simulink model "KUKAinv_Dynamics_coupled"  (R2021b)
settings: Solver=ode4  StartTime=0.0  StopTime=0.01  FixedStep=0.01  RelTol=1e-3
InitFcn:
  | % ************** Initiate forces
  | % f0=[0;0;0;0;0;0];
  | % f0=[0;0;0;0;0;0;0];
  | %f_0=[0;0;0];
  | %f_m=[0;1];
  | %f_e=[0;0;0;0;0;0];
  | % ************** Initiate states
  | %q_m=[0;0];
  | %q_dot_m=[0;0];
  | %P=[0;0;0];
  | %V_I0=[0;0;0];
  | % ************** Load main
  | %run(Main.m)
StopFcn:
  | %format long
  | %qddot=out.qddot.data(:,1)
  | %qddot_ref=out.qddot_ref.data(1,:)
values from neighbouring files (symbols this model uses):
  f_0 = [0;0;0;0;0;0]    [Initiate_FQ.m]    (also in Internal_KUKA_Main.m; KUKA_Main.m; Main.m = [0;0;0])
  f_e = [0;0;0;0;0;0]    [Initiate_FQ.m]    (also in Internal_KUKA_Main.m; KUKA_Main.m; Main.m)
  f_m = [0;0.1;0.2;0;0;0.01;0]    [Initiate_FQ.m]    (also in Internal_KUKA_Main.m = [0;0;0;0;0;0;0]; KUKA_Main.m = [0;0;0;0;0;0;0]; Main.m = [0;0])
  I0 = eye(3)*416.667    [Main.m]
  iota0 = eye(6,6)    [Internal_KUKA_Main.m]    (also in KUKA_Main.m; Main.m = [1 0 0; 0 1 0;zeros(3,3);0 0 1])
  m0 = robot.Bodies{1,n+1}.Mass    [Internal_KUKA_Main.m]    (also in KUKA_Main.m; Main.m = 100)
  mm = zeros(1,n)    [Internal_KUKA_Main.m]    (also in KUKA_Main.m; Main.m = [2 2])
  P0 = M0*V_I0+M0\M0m*q_dot_m    [Initiate_FQ.m]    (also in Internal_KUKA_Main.m; KUKA_Main.m)
  q_dot_m = [0;0;0;0;0;0;0]    [Initiate_FQ.m]    (also in Internal_KUKA_Main.m = [qdot1;qdot2;qdot3;qdot4;qdot5;qdot6;qdot7]; KUKA_Main.m = [qdot1;qdot2;qdot3;qdot4;qdot5;qdot6;qdot7]; Main.m = [0;0]; sendJointTorques.m = fread(t, 7, 'double'))
  q_m = [0.2;1.5;0.3;1.8;0.5;0.3;0.6]    [Initiate_FQ.m]    (also in Internal_KUKA_Main.m = [q_m1;q_m2;q_m3;q_m4;q_m5;q_m6;q_m7]; KUKA_Main.m = [q_m1;q_m2;q_m3;q_m4;q_m5;q_m6;q_m7]; Main.m = [0;0]; sendJointTorques.m = fread(t, 7, 'double'))
  sc_size = 0    [Internal_KUKA_Main.m]    (also in KUKA_Main.m = 1)
  V_I0 = [0;0;0;0;0;0]    [Initiate_FQ.m]    (also in Internal_KUKA_Main.m; KUKA_Main.m; Main.m = [0;0;0])
  X = [0 -x(3) x(2) ; x(3) 0 -x(1) ; -x(2) x(1) 0 ]    [skewsym.m]
  Xi_m = Xi_m(1:robot.n*6,1:robot.n)    [Internal_KUKA_Main.m]    (also in KUKA_Main.m)
  Xi_m_matrix = zeros(6*n,n)    [Internal_KUKA_Main.m]    (also in KUKA_Main.m; Main.m)
undefined symbols (not defined in the file or in its folder): g_cm, g_cm0, Im, m0_frak, m_diag, Y, Z
libraries: sm_lib x47, nesl_utility x41, robotcorelib x1
(part 1 of 2)
settings Model: Creator=Bmmog  LastModifiedBy=Bmmog
settings SimscapeCC: SimscapeLogType=all  SimscapeLogSimulationStatistics=on

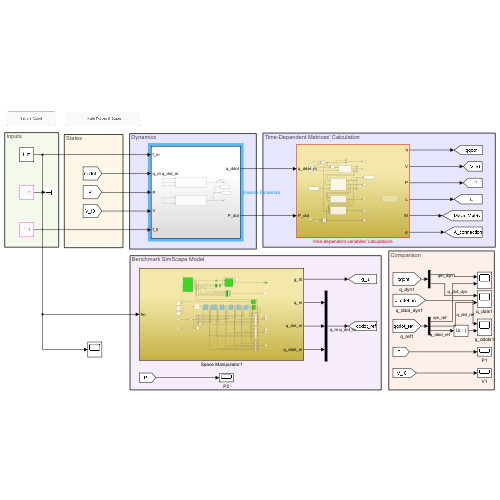
[thumbnail: Simulink's stored preview of the top-level diagram]
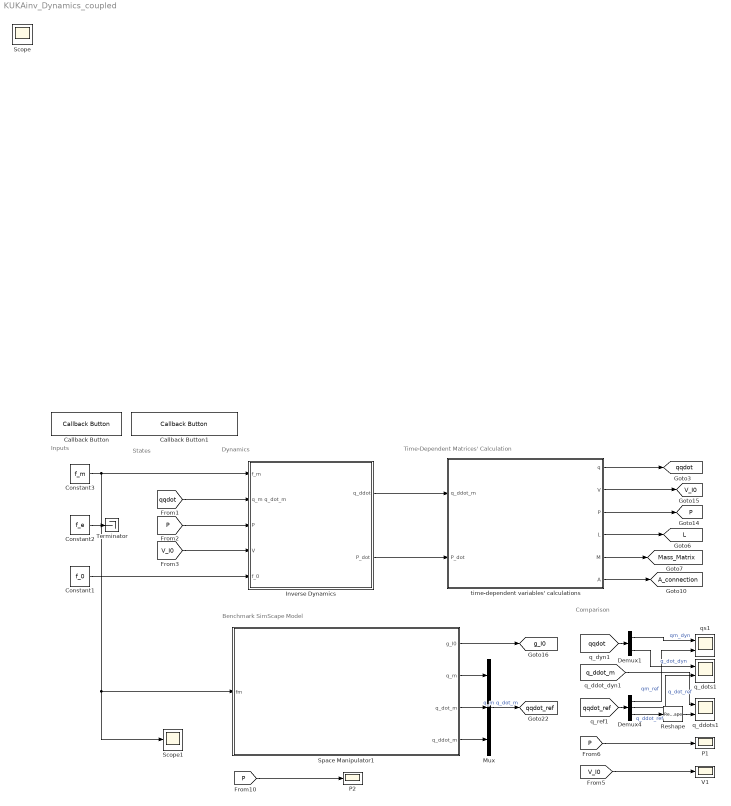
== system KUKAinv_Dynamics_coupled ==
  note: Dynamics
  note: Time-Dependent Matrices' Calculation
  note: States
  note: Comparison
  note: Inputs
  note: Benchmark SimScape Model
  Callback Button : CallbackButton  ButtonText=Initiate Robot
      settings: ClickFcn=Initiate_KUKA_inv
  Callback Button1 : CallbackButton  ButtonText=Initiate Forces & States
      settings: ClickFcn=Initiate_FQ
  Constant1 : Constant  Value=f_0  VectorParams1D=off
  Constant2 : Constant  Value=f_e  VectorParams1D=off
  Constant3 : Constant  Value=f_m  VectorParams1D=off
  Demux1 : Demux  Outputs=2
  Demux4 : Demux  Outputs=[7 7 7]
  Inverse Dynamics : Subsystem
  Mux : Mux  Inputs=3
  P1 : Scope
  P2 : Scope
  Reshape : Reshape
  Scope1 : Scope
  Space Manipulator1 : Subsystem
  Terminator : Terminator
  V1 : Scope
  q_ddots1 : Scope  NumInputPorts=2
  q_dots1 : Scope  NumInputPorts=2
  qs1 : Scope  NumInputPorts=2
  time-dependent variables' calculations : Subsystem
  Scope : Scope
  tag scope: A_connection=global, L=global, Mass_Matrix=global, P=global, V_I0=global, g_I0=global, qqdot=global, qqdot_ref=global
  wires:
  Demux4/3 -> Reshape/1  "q_ddot_ref"
  [qqdot] -> Inverse Dynamics/2(q_m q_dot_m)
  [qqdot_ref] -> Demux4/1
  Demux4/1 -> qs1/2  "qm_ref"
  Demux4/2 -> q_dots1/2  "q_dot_ref"
  [qqdot] -> Demux1/1
  Inverse Dynamics/1(q_ddot) -> time-dependent variables' calculations/1(q_ddot_m)
  Demux1/2 -> q_dots1/1  "q_dot_dyn"
  time-dependent variables' calculations/4(L) -> [L]
  time-dependent variables' calculations/5(M) -> [Mass_Matrix]
  time-dependent variables' calculations/1(q) -> [qqdot]
  Demux1/1 -> qs1/1  "qm_dyn"
  time-dependent variables' calculations/6(A) -> [A_connection]
  time-dependent variables' calculations/3(P) -> [P]
  time-dependent variables' calculations/2(V) -> [V_I0]
  Inverse Dynamics/2(P_dot) -> time-dependent variables' calculations/2(P_dot)
  [P] -> Inverse Dynamics/3(P)
  [V_I0] -> Inverse Dynamics/4(V)
  Constant1/1 -> Inverse Dynamics/5(f_0)
  [P] -> P1/1
  [V_I0] -> V1/1
  Space Manipulator1/3(q_dot_m) -> Mux/2
  Space Manipulator1/1(g_I0) -> [g_I0]
  Mux/1 -> [qqdot_ref]  "q_m q_dot_m"
  [P] -> P2/1
  Space Manipulator1/2(q_m) -> Mux/1
  Space Manipulator1/4(q_ddot_m) -> Mux/3
  Constant2/1 -> Terminator/1
  Constant3/1 -> Space Manipulator1/1(fm), Scope1/1, Inverse Dynamics/1(f_m)
  [q_ddot_m] -> q_ddots1/1
  Reshape/1 -> q_ddots1/2

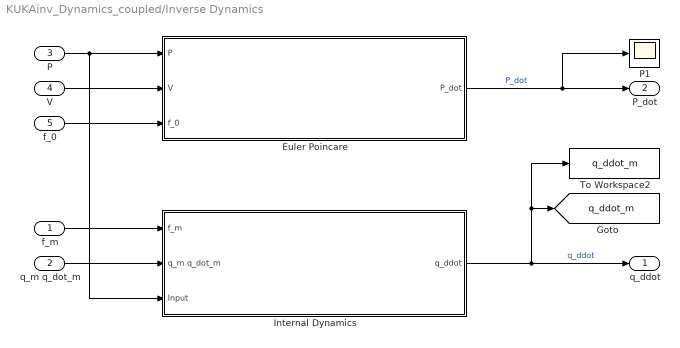
== system KUKAinv_Dynamics_coupled/Inverse Dynamics ==
  f_m : Inport
  q_m q_dot_m : Inport  Port=2
  P : Inport  Port=3
  V : Inport  Port=4
  f_0 : Inport  Port=5
  Euler Poincare : Subsystem
  Internal Dynamics : Subsystem
  P1 : Scope
  To Workspace2 : ToWorkspace  VariableName=q_ddot_m  SaveFormat=Timeseries  SampleTime=-1
  q_ddot : Outport
  P_dot : Outport  Port=2
  tag scope: q_ddot_m=global
  wires:
  f_m/1 -> Internal Dynamics/1(f_m)
  Internal Dynamics/1(q_ddot) -> To Workspace2/1, [q_ddot_m], q_ddot/1  "q_ddot"
  q_m q_dot_m/1 -> Internal Dynamics/2(q_m q_dot_m)
  Euler Poincare/1(P_dot) -> P1/1, P_dot/1  "P_dot"
  V/1 -> Euler Poincare/2(V)
  f_0/1 -> Euler Poincare/3(f_0)
  P/1 -> Internal Dynamics/3(Input), Euler Poincare/1(P)

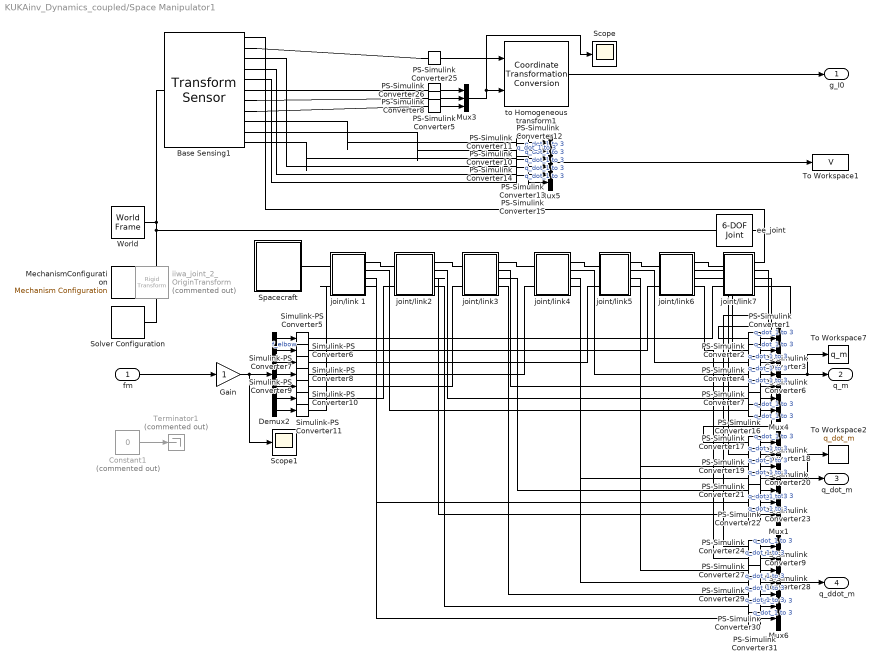
== system KUKAinv_Dynamics_coupled/Space Manipulator1 ==
  fm : Inport
  Base Sensing1 : sm_lib/Frames and Transforms/Transform Sensor  MeasurementFrame=Base  SenseAngle=off  SenseAxis=off  SenseAngle1=off  SenseAngle2=off  SenseAngle3=off  SenseQ=off  SenseR=on  SenseOmegaX=on  SenseOmegaY=on  SenseOmegaZ=on  SenseOmega1=off  SenseOmega2=off  SenseOmega3=off  SenseQDot=off  SenseRDot=off  SenseAlphaX=off  SenseAlphaY=off  SenseAlphaZ=off  SenseAlpha1=off  SenseAlpha2=off  SenseAlpha3=off  SenseQDDot=off  SenseRDDot=off  SenseX=on  SenseY=on  SenseZ=on  SenseRad=off  SenseAzim=off  SenseDist=off  SenseInc=off  SenseXDot=on  SenseYDot=on  SenseZDot=on  SenseRadDot=off  SenseAzimDot=off  SenseDistDot=off  SenseIncDot=off  SenseXDDot=off  SenseYDDot=off  SenseZDDot=off  SenseRadDDot=off  SenseAzimDDot=off  SenseDistDDot=off  SenseIncDDot=off
  Constant1 : Constant  Commented=on  Value=0
  Demux2 : Demux  Outputs=7
  Gain : Gain
  MechanismConfiguration : sm_lib/Utilities/Mechanism Configuration  UniformGravity=None  GravityVector=[0 0 0]  GravityUnits=m/s^2  LinearizationDelta=0.001  JointModeTransitionNonlinearIterations=2
  Mux1 : Mux  Inputs=7
  Mux3 : Mux  Inputs=3
  Mux4 : Mux  Inputs=7
  Mux5 : Mux  Inputs=6
  Mux6 : Mux  Inputs=7
  PS-Simulink Converter{1..31} (31 alike) : nesl_utility/PS-Simulink Converter  PhysicalDomain=network_engine_domain  SubClassName=ps_output  LeftPortType=input  RightPortType=output  PseudoPeriodic=off  Frequencies=[]  Unit=inherit  AffineConversion=off
      settings: SourceProductBaseCode=PW,SS
  Scope : Scope
  Scope1 : Scope
  Simulink-PS Converter{5..11} (7 alike) : nesl_utility/Simulink-PS Converter  PhysicalDomain=network_engine_domain  SubClassName=ps_input  LeftPortType=input  RightPortType=output  PseudoPeriodic=off  Frequencies=[]  NoiseDistribution=none  NoiseParameters=[]  Unit=1  AffineConversion=off  FilteringAndDerivatives=provide  SimscapeFilterOrder=1  InputFilterTimeConstant=0.001  UdotUserProvided=0
      settings: SourceProductBaseCode=PW,SS
  Solver Configuration : nesl_utility/Solver Configuration  PhysicalDomain=network_engine_domain  SubClassName=solver  LeftPortType=input  RightPortType=generic  Tones=[]  Harmonics=[]  SimulateNoise=off  Profile=off  UseLocalSampling=off  EnableSwitchedLinearOptims=on  FrequencyDomain=off  UseCCode=off  RelTol=0.001  AbsTol=0.001  MinStep=1e-09  ToWorkspace=off  RevertToSquareIcSolve=off  NumHomotopyIterations=100  PhasorMode=off  PhasorModeNumHarmonics=1  DoDC=off  ResidualTolerance=1e-09  UseLocalSolver=on  LocalSolverChoice=NE_BACKWARD_EULER_ADVANCER  LocalSolverSampleTime=0.001  DoFixedCost=on  MaxNonlinIter=3  MaxModeIter=2  ComputeImpulses=off  ImpulseIterations=2  LinearAlgebra=auto  EquationFormulation=NE_TIME_EF  DelaysMemoryBudget=1024  AutomaticFiltering=on  FilteringTimeConstant=0.001  PartitionStorageMethod=AS_NEEDED  PartitionMemoryBudget=1024  PartitionMethod=ROBUST
      settings: SourceProductBaseCode=PW,SS
  Spacecraft : Subsystem
  Terminator1 : Terminator  Commented=on
  To Workspace1 : ToWorkspace  VariableName=V  SaveFormat=Timeseries  SampleTime=-1
  To Workspace2 : ToWorkspace  VariableName=q_dot_m  SampleTime=-1
  To Workspace7 : ToWorkspace  VariableName=q_m  SampleTime=-1
  World : sm_lib/Frames and Transforms/World Frame
  ee_joint : sm_lib/Joints/6-DOF Joint  JointMode=Normal  SenseConstraintForce=off  SenseConstraintForceX=off  SenseConstraintForceY=off  SenseConstraintForceZ=off  SenseConstraintTorque=off  SenseConstraintTorqueX=off  SenseConstraintTorqueY=off  SenseConstraintTorqueZ=off  SenseTotalForce=off  SenseTotalForceX=off  SenseTotalForceY=off  SenseTotalForceZ=off  SenseTotalTorque=off  SenseTotalTorqueX=off  SenseTotalTorqueY=off  SenseTotalTorqueZ=off  CompositeWrenchDir=FollowerOnBase  CompositeWrenchFrame=BaseFrame  PxEquilibriumPosition=0  PxEquilibriumPositionUnits=m  PxSpringStiffness=0  PxSpringStiffnessUnits=N/m  PxDampingCoefficient=0  PxDampingCoefficientUnits=N/(m/s)  PxTorqueActuationMode=NoTorque  PxMotionActuationMode=ComputedMotion  PxSensePosition=off  PxSenseVelocity=off  PxSenseAcceleration=off  PxSenseTorqueForce=off  PxSenseLowerLimitTorqueForce=off  PxSenseUpperLimitTorqueForce=off  PxLowerLimitSpecify=off  PxLowerLimitBound=-1  PxLowerLimitBoundUnits=m  PxLowerLimitStiffness=1e6  PxLowerLimitStiffnessUnits=N/m  PxLowerLimitDamping=1e3  PxLowerLimitDampingUnits=N/(m/s)  PxLowerLimitTransitionRegionWidth=1e-4  PxLowerLimitTransitionRegionWidthUnits=m  PxUpperLimitSpecify=off  PxUpperLimitBound=1  PxUpperLimitBoundUnits=m  PxUpperLimitStiffness=1e6  PxUpperLimitStiffnessUnits=N/m  PxUpperLimitDamping=1e3  PxUpperLimitDampingUnits=N/(m/s)  PxUpperLimitTransitionRegionWidth=1e-4  PxUpperLimitTransitionRegionWidthUnits=m  PxPositionTargetSpecify=off  PxPositionTargetPriority=High  PxPositionTargetValue=0  PxPositionTargetValueUnits=m  PxVelocityTargetSpecify=on  PxVelocityTargetPriority=High  PxVelocityTargetValue=V_I0(1)  PxVelocityTargetValueUnits=m/s  PyEquilibriumPosition=0  PyEquilibriumPositionUnits=m  PySpringStiffness=0  PySpringStiffnessUnits=N/m  PyDampingCoefficient=0  PyDampingCoefficientUnits=N/(m/s)  PyTorqueActuationMode=NoTorque  PyMotionActuationMode=ComputedMotion  PySensePosition=off  PySenseVelocity=off  PySenseAcceleration=off  PySenseTorqueForce=off  PySenseLowerLimitTorqueForce=off  PySenseUpperLimitTorqueForce=off  PyLowerLimitSpecify=off  PyLowerLimitBound=-1  PyLowerLimitBoundUnits=m  PyLowerLimitStiffness=1e6  PyLowerLimitStiffnessUnits=N/m  PyLowerLimitDamping=1e3  PyLowerLimitDampingUnits=N/(m/s)  PyLowerLimitTransitionRegionWidth=1e-4  PyLowerLimitTransitionRegionWidthUnits=m  PyUpperLimitSpecify=off  PyUpperLimitBound=1  PyUpperLimitBoundUnits=m  PyUpperLimitStiffness=1e6  PyUpperLimitStiffnessUnits=N/m  PyUpperLimitDamping=1e3  PyUpperLimitDampingUnits=N/(m/s)  PyUpperLimitTransitionRegionWidth=1e-4  PyUpperLimitTransitionRegionWidthUnits=m  PyPositionTargetSpecify=off  PyPositionTargetPriority=High  PyPositionTargetValue=0  PyPositionTargetValueUnits=m  PyVelocityTargetSpecify=on  PyVelocityTargetPriority=High  PyVelocityTargetValue=V_I0(2)  PyVelocityTargetValueUnits=m/s  PzEquilibriumPosition=0  PzEquilibriumPositionUnits=m  PzSpringStiffness=0  PzSpringStiffnessUnits=N/m  PzDampingCoefficient=0  PzDampingCoefficientUnits=N/(m/s)  PzTorqueActuationMode=NoTorque  PzMotionActuationMode=ComputedMotion  PzSensePosition=off  PzSenseVelocity=off  PzSenseAcceleration=off  PzSenseTorqueForce=off  PzSenseLowerLimitTorqueForce=off  PzSenseUpperLimitTorqueForce=off  PzLowerLimitSpecify=off  PzLowerLimitBound=-1  PzLowerLimitBoundUnits=m  PzLowerLimitStiffness=1e6  PzLowerLimitStiffnessUnits=N/m  PzLowerLimitDamping=1e3  PzLowerLimitDampingUnits=N/(m/s)  PzLowerLimitTransitionRegionWidth=1e-4  PzLowerLimitTransitionRegionWidthUnits=m  PzUpperLimitSpecify=off  PzUpperLimitBound=1  PzUpperLimitBoundUnits=m  PzUpperLimitStiffness=1e6  PzUpperLimitStiffnessUnits=N/m  PzUpperLimitDamping=1e3  PzUpperLimitDampingUnits=N/(m/s)  PzUpperLimitTransitionRegionWidth=1e-4  PzUpperLimitTransitionRegionWidthUnits=m  PzPositionTargetSpecify=off  PzPositionTargetPriority=High  PzPositionTargetValue=0  PzPositionTargetValueUnits=m  PzVelocityTargetSpecify=on  PzVelocityTargetPriority=High  PzVelocityTargetValue=V_I0(3)  PzVelocityTargetValueUnits=m/s  SphDefPosRotationMethod=None  SphDefPosRotationAngleUnits=deg  SphDefPosRotationStandardAxis=+Z  SphDefPosRotationAngle=0.0  SphDefPosRotationArbitraryAxis=[0 0 1]  SphDefPosFollAlignAxisA=+X  SphDefPosBaseAlignAxisA=+Y  SphDefPosFollAlignAxisB=+Y  SphDefPosBaseAlignAxisB=+Z  SphDefPosRotationSequenceAxes=FollowerAxes  SphDefPosRotationSequence=XYX  SphDefPosRotationSequenceAngles=[0 0 0]  SphDefPosRotationSequenceAnglesUnits=deg  SphDefPosRotationMatrix=[1 0 0; 0 1 0; 0 0 1]  SphEqPosRotationMethod=None  SphEqPosRotationAngleUnits=deg  SphEqPosRotationStandardAxis=+Z  SphEqPosRotationAngle=0.0  SphEqPosRotationArbitraryAxis=[0 0 1]  SphEqPosFollAlignAxisA=+X  SphEqPosBaseAlignAxisA=+Y  SphEqPosFollAlignAxisB=+Y  SphEqPosBaseAlignAxisB=+Z  SphEqPosRotationSequenceAxes=FollowerAxes  SphEqPosRotationSequence=XYX  SphEqPosRotationSequenceAngles=[0 0 0]  SphEqPosRotationSequenceAnglesUnits=deg  SphEqPosRotationMatrix=[1 0 0; 0 1 0; 0 0 1]  SphSpringStiffness=0  SphSpringStiffnessUnits=N*m/deg  SphDampingCoefficient=0  SphDampingCoefficientUnits=N*m/(deg/s)  SphActuateTorqueX=off  SphActuateTorqueY=off  SphActuateTorqueZ=off  SphActuateTorque=off  SphTorqueActuationMode=NoTorque  SphMotionActuationMode=ComputedMotion  SphActuationFrame=BaseFrame  SphSensePosition=off  SphSenseVelocityX=off  SphSenseVelocityY=off  SphSenseVelocityZ=off  SphSenseVelocity=off  SphSenseAccelerationX=off  SphSenseAccelerationY=off  SphSenseAccelerationZ=off  SphSenseAcceleration=off  SphSenseTorqueX=off  SphSenseTorqueY=off  SphSenseTorqueZ=off  SphSenseTorqueForce=off  SphSenseLowerLimitTorqueMag=off  SphSenseUpperLimitTorqueMag=off  SphSensingFrame=BaseFrame  SphLowerLimitSpecify=off  SphLowerLimitBound=15  SphLowerLimitBoundUnits=deg  SphLowerLimitStiffness=1e4  SphLowerLimitStiffnessUnits=N*m/deg  SphLowerLimitDamping=10  SphLowerLimitDampingUnits=N*m/(deg/s)  SphLowerLimitTransitionRegionWidth=0.1  SphLowerLimitTransitionRegionWidthUnits=deg  SphUpperLimitSpecify=off  SphUpperLimitBound=45  SphUpperLimitBoundUnits=deg  SphUpperLimitStiffness=1e4  SphUpperLimitStiffnessUnits=N*m/deg  SphUpperLimitDamping=10  SphUpperLimitDampingUnits=N*m/(deg/s)  SphUpperLimitTransitionRegionWidth=0.1  SphUpperLimitTransitionRegionWidthUnits=deg  SphPositionTargetRotationMethod=RotationSequence  SphPositionTargetRotationAngleUnits=deg  SphPositionTargetRotationStandardAxis=+Z  SphPositionTargetRotationAngle=0.0  SphPositionTargetRotationArbitraryAxis=[0 0 1]  SphPositionTargetFollAlignAxisA=+X  SphPositionTargetBaseAlignAxisA=+Y  SphPositionTargetFollAlignAxisB=+Y  SphPositionTargetBaseAlignAxisB=+Z  SphPositionTargetRotationSequenceAxes=FollowerAxes  SphPositionTargetRotationSequence=ZYX  SphPositionTargetRotationSequenceAngles=[0 0 0]  SphPositionTargetRotationSequenceAnglesUnits=deg  SphPositionTargetRotationMatrix=[1 0 0; 0 1 0; 0 0 1]  SphPositionTargetSpecify=off  SphPositionTargetPriority=High  SphVelocityTargetValue=[V_I0(4) V_I0(5) V_I0(6)]  SphVelocityTargetValueUnits=rad/s  SphVelocityTargetSpecify=on  SphVelocityTargetPriority=High  SphVelocityTargetInFollowerFrame=on
  iiwa_joint_2_OriginTransform : sm_lib/Frames and Transforms/Rigid Transform  Commented=on  TranslationMethod=Cartesian  TranslationStandardOffset=0  TranslationLengthUnit=m  TranslationStandardAxis=+Z  TranslationCartesianOffset=g_cm(1:3,4,7)'  TranslationROffset=0  TranslationROffsetUnits=m  TranslationZOffset=0  TranslationZOffsetUnits=m  TranslationThetaOffset=0  TranslationThetaOffsetUnits=deg  RotationMethod=RotationMatrix  RotationAngleUnits=deg  RotationStandardAxis=+Z  RotationAngle=0.0  RotationArbitraryAxis=[0 0 1]  FollAlignAxisA=+X  BaseAlignAxisA=+Y  FollAlignAxisB=+Y  BaseAlignAxisB=+Z  RotationSequenceAxes=BaseAxes  RotationSequence=XYZ  RotationSequenceAngles=[1.57079632679, 0, 3.14159265359]  RotationSequenceAnglesUnits=rad  RotationMatrix=g_cm(1:3,1:3,7)
  join/link 1 : Subsystem
  joint/link2 : Subsystem
  joint/link3 : Subsystem
  joint/link4 : Subsystem
  joint/link5 : Subsystem
  joint/link6 : Subsystem
  joint/link7 : Subsystem
  to Homogeneous transform1 : robotcorelib/Coordinate Transformation Conversion  InputRepresentation=Rotation Matrix  InputEulerSequence=ZYX  ShowTrVecInputPort=on  OutputRepresentation=Homogeneous Transformation  OutputEulerSequence=ZYX  ShowTrVecOutputPort=on  SimulateUsing=Interpreted execution
      settings: SourceProductBaseCode=NV,RO,RR,UV
  g_I0 : Outport
  q_m : Outport  Port=2
  q_dot_m : Outport  Port=3
  q_ddot_m : Outport  Port=4
  wires:
  Demux2/1 -> Simulink-PS Converter5/1
  Demux2/3 -> Simulink-PS Converter7/1
  PS-Simulink Converter15/1 -> Mux5/6  "q_dot_1 to 3"
  PS-Simulink Converter10/1 -> Mux5/3  "q_dot_1 to 3"
  fm/1 -> Gain/1
  PS-Simulink Converter25/1 -> to Homogeneous transform1/1
  Gain/1 -> Scope1/1, Demux2/1
  Mux5/1 -> To Workspace1/1
  PS-Simulink Converter8/1 -> Mux3/3
  Mux3/1 -> Scope/1, to Homogeneous transform1/2
  PS-Simulink Converter12/1 -> Mux5/2  "q_dot_1 to 3"
  to Homogeneous transform1/1 -> g_I0/1
  PS-Simulink Converter13/1 -> Mux5/4  "q_dot_1 to 3"
  PS-Simulink Converter26/1 -> Mux3/1
  Demux2/7 -> Simulink-PS Converter11/1
  PS-Simulink Converter14/1 -> Mux5/5  "q_dot_1 to 3"
  Demux2/4 -> Simulink-PS Converter8/1
  PS-Simulink Converter11/1 -> Mux5/1  "q_dot_1 to 3"
  PS-Simulink Converter5/1 -> Mux3/2
  Demux2/6 -> Simulink-PS Converter10/1
  Constant1/1 -> Terminator1/1
  Demux2/2 -> Simulink-PS Converter6/1  "f_elbow"
  Demux2/5 -> Simulink-PS Converter9/1
  PS-Simulink Converter27/1 -> Mux6/3  "q_dot_1 to 3"
  PS-Simulink Converter1/1 -> Mux4/1  "q_dot_1 to 3"
  PS-Simulink Converter6/1 -> Mux4/5  "q_dot_1 to 3"
  PS-Simulink Converter30/1 -> Mux6/6  "q_dot_1 to 3"
  PS-Simulink Converter3/1 -> Mux4/3  "q_dot_1 to 3"
  PS-Simulink Converter18/1 -> Mux1/2  "q_dot_1 to 3"
  PS-Simulink Converter31/1 -> Mux6/7  "q_dot_1 to 3"
  PS-Simulink Converter9/1 -> Mux6/2  "q_dot_1 to 3"
  PS-Simulink Converter7/1 -> Mux4/6  "q_dot_1 to 3"
  PS-Simulink Converter2/1 -> Mux4/2  "q_dot_1 to 3"
  PS-Simulink Converter4/1 -> Mux4/4  "q_dot_1 to 3"
  PS-Simulink Converter21/1 -> Mux1/5  "q_dot_1 to 3"
  PS-Simulink Converter23/1 -> Mux1/7  "q_dot_1 to 3"
  PS-Simulink Converter16/1 -> Mux4/7  "q_dot_1 to 3"
  PS-Simulink Converter28/1 -> Mux6/4  "q_dot_1 to 3"
  Mux4/1 -> q_m/1, To Workspace7/1
  Mux1/1 -> q_dot_m/1, To Workspace2/1
  PS-Simulink Converter24/1 -> Mux6/1  "q_dot_1 to 3"
  Mux6/1 -> q_ddot_m/1
  PS-Simulink Converter20/1 -> Mux1/4  "q_dot_1 to 3"
  PS-Simulink Converter29/1 -> Mux6/5  "q_dot_1 to 3"
  PS-Simulink Converter22/1 -> Mux1/6  "q_dot_1 to 3"
  PS-Simulink Converter17/1 -> Mux1/1  "q_dot_1 to 3"
  PS-Simulink Converter19/1 -> Mux1/3  "q_dot_1 to 3"
  connections:
  ee_joint/LConn1 -- MechanismConfiguration/RConn1 -- Solver Configuration/RConn1 -- World/RConn1 -- Base Sensing1/LConn1
  ee_joint/RConn1 -- Base Sensing1/RConn1 -- joint/link7/RConn1
  joint/link4/LConn1 -- joint/link3/RConn1
  Base Sensing1/RConn10 -- PS-Simulink Converter12/LConn1
  Simulink-PS Converter9/RConn1 -- joint/link3/LConn2
  Simulink-PS Converter8/RConn1 -- joint/link4/LConn2
  Base Sensing1/RConn2 -- PS-Simulink Converter25/LConn1
  joint/link5/LConn1 -- joint/link4/RConn1
  Base Sensing1/RConn5 -- PS-Simulink Converter15/LConn1
  Base Sensing1/RConn7 -- PS-Simulink Converter5/LConn1
  joint/link6/LConn1 -- joint/link5/RConn1
  Base Sensing1/RConn11 -- PS-Simulink Converter10/LConn1
  Base Sensing1/RConn3 -- PS-Simulink Converter13/LConn1
  Simulink-PS Converter5/RConn1 -- joint/link7/LConn2
  Base Sensing1/RConn4 -- PS-Simulink Converter14/LConn1
  Base Sensing1/RConn9 -- PS-Simulink Converter11/LConn1
  Base Sensing1/RConn8 -- PS-Simulink Converter8/LConn1
  Base Sensing1/RConn6 -- PS-Simulink Converter26/LConn1
  Simulink-PS Converter7/RConn1 -- joint/link5/LConn2
  joint/link6/RConn3 -- PS-Simulink Converter18/LConn1
  joint/link6/RConn4 -- PS-Simulink Converter9/LConn1
  joint/link5/RConn2 -- PS-Simulink Converter3/LConn1
  joint/link5/RConn3 -- PS-Simulink Converter19/LConn1
  joint/link5/RConn4 -- PS-Simulink Converter27/LConn1
  joint/link4/RConn2 -- PS-Simulink Converter4/LConn1
  joint/link4/RConn3 -- PS-Simulink Converter20/LConn1
  joint/link4/RConn4 -- PS-Simulink Converter28/LConn1
  joint/link3/RConn2 -- PS-Simulink Converter6/LConn1
  joint/link3/RConn3 -- PS-Simulink Converter21/LConn1
  joint/link3/RConn4 -- PS-Simulink Converter29/LConn1
  joint/link6/RConn1 -- joint/link7/LConn1
  joint/link6/RConn2 -- PS-Simulink Converter2/LConn1
  joint/link6/LConn2 -- Simulink-PS Converter6/RConn1
  joint/link7/RConn2 -- PS-Simulink Converter1/LConn1
  joint/link7/RConn3 -- PS-Simulink Converter17/LConn1
  joint/link7/RConn4 -- PS-Simulink Converter24/LConn1
  join/link 1/LConn2 -- Simulink-PS Converter11/RConn1
  join/link 1/LConn1 -- Spacecraft/RConn1
  join/link 1/RConn1 -- joint/link2/LConn1
  Simulink-PS Converter10/RConn1 -- joint/link2/LConn2
  joint/link3/LConn1 -- joint/link2/RConn1
  join/link 1/RConn2 -- PS-Simulink Converter16/LConn1
  joint/link2/RConn3 -- PS-Simulink Converter23/LConn1
  PS-Simulink Converter7/LConn1 -- joint/link2/RConn2
  join/link 1/RConn3 -- PS-Simulink Converter22/LConn1
  joint/link2/RConn4 -- PS-Simulink Converter30/LConn1
  join/link 1/RConn4 -- PS-Simulink Converter31/LConn1

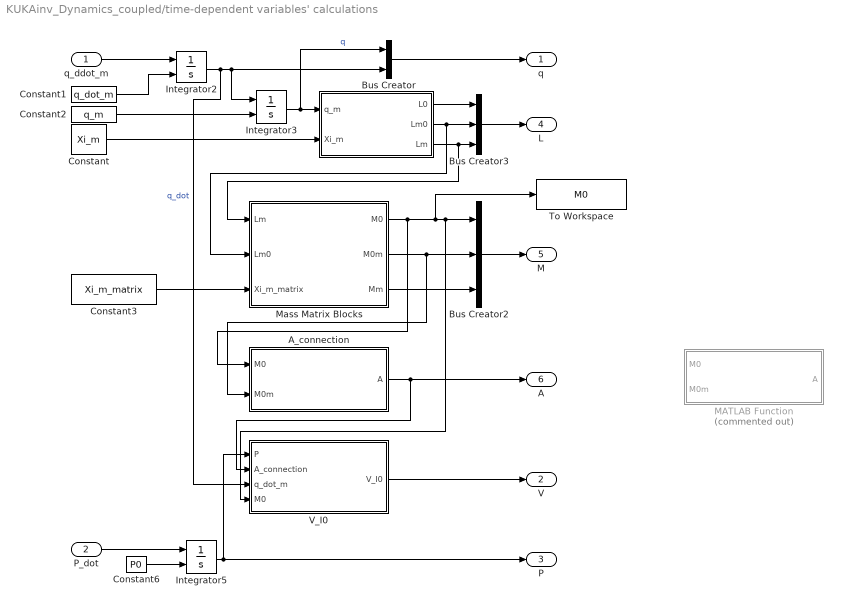
== system KUKAinv_Dynamics_coupled/time-dependent variables' calculations ==
  q_ddot_m : Inport
  P_dot : Inport  Port=2
  " " : MATLAB Function  TreatAsAtomicUnit=on
  A_connection : Subsystem
  Bus Creator : BusCreator  Inputs=2
  Bus Creator2 : BusCreator  Inputs=3
  Bus Creator3 : BusCreator  Inputs=3
  Constant : Constant  Value=Xi_m
  Constant1 : Constant  Value=q_dot_m  VectorParams1D=off
  Constant2 : Constant  Value=q_m  VectorParams1D=off
  Constant3 : Constant  Value=Xi_m_matrix
  Constant6 : Constant  Value=P0  VectorParams1D=off
  Integrator2 : Integrator  InitialConditionSource=external  InitialCondition=q_dot_m
  Integrator3 : Integrator  InitialConditionSource=external
  Integrator5 : Integrator  InitialConditionSource=external  ContinuousStateAttributes='momentum'
  MATLAB Function : MATLAB Function  Commented=on  TreatAsAtomicUnit=on
  Mass Matrix Blocks : Subsystem
  To Workspace : ToWorkspace  VariableName=M0  SaveFormat=Timeseries  SampleTime=-1
  V_I0 : MATLAB Function  TreatAsAtomicUnit=on
  q : Outport
  V : Outport  Port=2
  P : Outport  Port=3
  L : Outport  Port=4
  M : Outport  Port=5
  A : Outport  Port=6
  wires:
  q_ddot_m/1 -> Integrator2/1
  " "/3(Lm) -> Bus Creator3/3, Mass Matrix Blocks/1(Lm)
  Constant3/1 -> Mass Matrix Blocks/3(Xi_m_matrix)
  Constant/1 -> " "/2(Xi_m)
  Constant1/1 -> Integrator2/2
  Constant2/1 -> Integrator3/2
  Bus Creator/1 -> q/1
  Integrator3/1 -> Bus Creator/1, " "/1(q_m)  "q"
  Integrator2/1 -> V_I0/3(q_dot_m), Bus Creator/2, Integrator3/1  "q_dot"
  V_I0/1(V_I0) -> V/1
  Integrator5/1 -> V_I0/1(P), P/1
  P_dot/1 -> Integrator5/1
  Constant6/1 -> Integrator5/2
  Mass Matrix Blocks/3(Mm) -> Bus Creator2/3
  " "/2(Lm0) -> Mass Matrix Blocks/2(Lm0), Bus Creator3/2
  " "/1(L0) -> Bus Creator3/1
  Bus Creator3/1 -> L/1
  Bus Creator2/1 -> M/1
  Mass Matrix Blocks/1(M0) -> A_connection/1(M0), To Workspace/1, V_I0/4(M0), Bus Creator2/1
  Mass Matrix Blocks/2(M0m) -> A_connection/2(M0m), Bus Creator2/2
  A_connection/1(A) -> V_I0/2(A_connection), A/1

== system KUKAinv_Dynamics_coupled/Inverse Dynamics/Euler Poincare ==
  P : Inport
  V : Inport  Port=2
  f_0 : Inport  Port=3
  Add : Sum
  Constant1 : Constant  Commented=on  Value=eye(6,6)
  MATLAB Function : MATLAB Function  Commented=on  TreatAsAtomicUnit=on
  Matrix Multiply : Product  Multiplication=Matrix(*)
  adj_low_tilde : MATLAB Function  TreatAsAtomicUnit=on
  P_dot : Outport
  wires:
  P/1 -> adj_low_tilde/1(P)
  V/1 -> Matrix Multiply/2
  Matrix Multiply/1 -> Add/1
  f_0/1 -> Add/2
  Add/1 -> P_dot/1
  adj_low_tilde/1(adj_low_tilde) -> Matrix Multiply/1

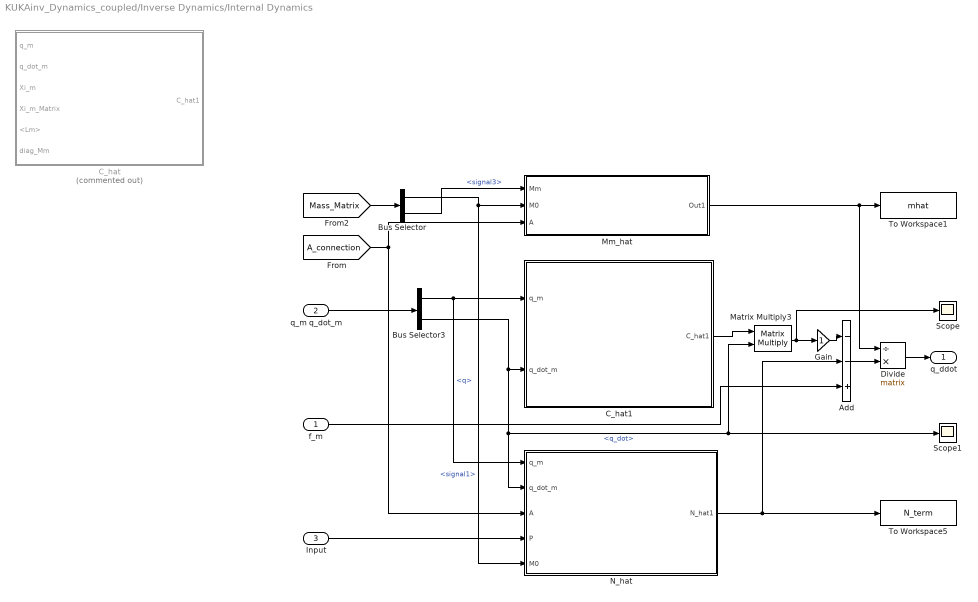
== system KUKAinv_Dynamics_coupled/Inverse Dynamics/Internal Dynamics ==
  f_m : Inport
  q_m q_dot_m : Inport  Port=2
  Input : Inport  Port=3
  Add : Sum  Inputs=--+
  Bus Selector : BusSelector  OutputSignals=signal1,signal3
  Bus Selector3 : BusSelector  OutputSignals=q,q_dot
  C_hat : Subsystem  Commented=on
  C_hat1 : Subsystem
  Divide : Product  Inputs=/*  Multiplication=Matrix(*)
  Gain : Gain
  Matrix Multiply3 : Product  Multiplication=Matrix(*)
  Mm_hat : Subsystem
  N_hat : Subsystem
  Scope : Scope
  Scope1 : Scope
  To Workspace1 : ToWorkspace  VariableName=mhat  SaveFormat=Timeseries  SampleTime=-1
  To Workspace5 : ToWorkspace  VariableName=N_term  SaveFormat=Timeseries  SampleTime=-1
  q_ddot : Outport
  wires:
  f_m/1 -> Add/3
  C_hat1/1(C_hat1) -> Matrix Multiply3/1
  Matrix Multiply3/1 -> Scope/1, Gain/1
  Bus Selector3/2 -> N_hat/2(q_dot_m), Scope1/1, Matrix Multiply3/2, C_hat1/2(q_dot_m)  "<q_dot>"
  q_m q_dot_m/1 -> Bus Selector3/1
  Divide/1 -> q_ddot/1
  Bus Selector3/1 -> N_hat/1(q_m), C_hat1/1(q_m)  "<q>"
  Add/1 -> Divide/2
  [Mass_Matrix] -> Bus Selector/1
  Gain/1 -> Add/1
  Bus Selector/1 -> N_hat/5(M0), Mm_hat/2(M0)  "<signal1>"
  [A_connection] -> Mm_hat/3(A), N_hat/3(A)
  Input/1 -> N_hat/4(P)
  N_hat/1(N_hat1) -> To Workspace5/1, Add/2
  Mm_hat/1(Out1) -> Divide/1, To Workspace1/1
  Bus Selector/2 -> Mm_hat/1(Mm)  "<signal3>"

== system KUKAinv_Dynamics_coupled/Space Manipulator1/Spacecraft ==
  Base1 : sm_lib/Body Elements/Brick Solid  GraphicAmbientColor=[0.15 0.15 0.15 1.0]  BasedOnType=Mass  BrickDimensions=[sc_size,sc_size,sc_size]  BrickDimensionUnits=m  CenterOfMass=[0 0 0]  CenterOfMassUnits=m  GraphicDiffuseColor=[0.5 0.5 0.5]  Density=1000  DensityUnits=kg/m^3  DoExposeReferenceFrame=on  GraphicEmissiveColor=[0.0 0.0 0.0 1.0]  ExportEntireGeometry=off  SerializedFrames=<Frames><Frame><Id>Frame1</Id><Value><Name>F1</Name><Origin><Source>GeometricFeature</Source><FeatureName>+z surface</FeatureName></Origin><PrimaryAxis><DefinedDirection>+X</DefinedDirection><Source>ReferenceFrame</Source><SourceDirection>+X</SourceDirection><FeatureName></FeatureName></PrimaryAxis><SecondaryAxis><DefinedDirection>+Z</DefinedDirection><Source>ReferenceFrame</Source><SourceDirection>+Z</SourceDirection><FeatureName></FeatureName></SecondaryAxis></Value></Frame></Frames>  MarkerShape=Sphere  MarkerSize=10  GraphicType=FromGeometry  InertiaType=Custom  Mass=0  MassUnits=kg  MomentsOfInertia=[0 0 0]  MomentsOfInertiaUnits=kg*m^2  GraphicOpacity=1.0  ProductsOfInertia=[0 0 0]  ProductsOfInertiaUnits=kg*m^2  GraphicShininess=75  GraphicSpecularColor=[0.5 0.5 0.5 1.0]  GraphicVisPropType=SimpleVisualProperties
  Base2 : sm_lib/Body Elements/Brick Solid  Commented=on  GraphicAmbientColor=[0.15 0.15 0.15 1.0]  BasedOnType=Mass  BrickDimensions=[sc_size,sc_size,sc_size]  BrickDimensionUnits=m  CenterOfMass=[0 0 0]  CenterOfMassUnits=m  GraphicDiffuseColor=[0.5 0.5 0.5]  Density=1000  DensityUnits=kg/m^3  DoExposeReferenceFrame=on  GraphicEmissiveColor=[0.0 0.0 0.0 1.0]  ExportEntireGeometry=off  SerializedFrames=<Frames><Frame><Id>Frame1</Id><Value><Name>F1</Name><Origin><Source>GeometricFeature</Source><FeatureName>+z surface</FeatureName></Origin><PrimaryAxis><DefinedDirection>+X</DefinedDirection><Source>ReferenceFrame</Source><SourceDirection>+X</SourceDirection><FeatureName></FeatureName></PrimaryAxis><SecondaryAxis><DefinedDirection>+Z</DefinedDirection><Source>ReferenceFrame</Source><SourceDirection>+Z</SourceDirection><FeatureName></FeatureName></SecondaryAxis></Value></Frame></Frames>  MarkerShape=Sphere  MarkerSize=10  GraphicType=FromGeometry  InertiaType=CalculateFromGeometry  Mass=10  MassUnits=kg  MomentsOfInertia=[0 0 0]  MomentsOfInertiaUnits=kg*m^2  GraphicOpacity=1.0  ProductsOfInertia=[0 0 0]  ProductsOfInertiaUnits=kg*m^2  GraphicShininess=75  GraphicSpecularColor=[0.5 0.5 0.5 1.0]  GraphicVisPropType=SimpleVisualProperties
  Inertia : sm_lib/Body Elements/Inertia  InertiaType=Custom  Mass=mm(7)  MassUnits=kg  CenterOfMass=[0, 0, 0]  CenterOfMassUnits=m  MomentsOfInertia=[Im(1,1,7) Im(2,2,7) Im(3,3,7)]  MomentsOfInertiaUnits=kg*m^2  ProductsOfInertia=[Im(3,2,7) Im(3,1,7) Im(2,1,7)]  ProductsOfInertiaUnits=kg*m^2  GraphicType=None  MarkerShape=Inertia  MarkerSize=20  GraphicVisPropType=SimpleVisualProperties  GraphicDiffuseColor=[0.5 0.5 0.5]  GraphicSpecularColor=[0.5 0.5 0.5 1.0]  GraphicAmbientColor=[0.15 0.15 0.15 1.0]  GraphicEmissiveColor=[0.0 0.0 0.0 1.0]  GraphicShininess=75  GraphicOpacity=1.0
  Visual : sm_lib/Body Elements/File Solid  Commented=on  ExtGeomFileName=iiwa_description/meshes/iiwa7/visual/link_1.stl  UnitType=Custom  ExtGeomFileUnits=m  StepReaderType=HEX  ExportConvexHullGeometry=off  InertiaType=Custom  Mass=0  MassUnits=kg  CenterOfMass=[0, 0, 0]  CenterOfMassUnits=m  MomentsOfInertia=[0, 0, 0]  MomentsOfInertiaUnits=kg*m^2  ProductsOfInertia=[0, 0, 0]  ProductsOfInertiaUnits=kg*m^2  BasedOnType=DensityFromFile  Density=1000  DensityUnits=kg/m^3  DoExposeReferenceFrame=on  SerializedFrames=<Frames/>  GraphicType=FromGeometry  MarkerShape=Sphere  MarkerSize=10  GraphicVisPropType=SimpleVisualProperties  GraphicDiffuseColor=[1, 0.423529411765, 0.0392156862745]  GraphicSpecularColor=[0.5 0.5 0.5 1.0]  GraphicAmbientColor=[0.15 0.15 0.15 1.0]  GraphicEmissiveColor=[0.0 0.0 0.0 1.0]  GraphicShininess=75  GraphicOpacity=1
  VisualOriginTransform : sm_lib/Frames and Transforms/Rigid Transform  TranslationMethod=Cartesian  TranslationStandardOffset=0  TranslationLengthUnit=m  TranslationStandardAxis=+Z  TranslationCartesianOffset=[0, 0, 0]  TranslationROffset=0  TranslationROffsetUnits=m  TranslationZOffset=0  TranslationZOffsetUnits=m  TranslationThetaOffset=0  TranslationThetaOffsetUnits=deg  RotationMethod=RotationSequence  RotationAngleUnits=deg  RotationStandardAxis=+Z  RotationAngle=0.0  RotationArbitraryAxis=[0 0 1]  FollAlignAxisA=+X  BaseAlignAxisA=+Y  FollAlignAxisB=+Y  BaseAlignAxisB=+Z  RotationSequenceAxes=BaseAxes  RotationSequence=XYZ  RotationSequenceAngles=[0, 0, 0]  RotationSequenceAnglesUnits=rad  RotationMatrix=[1 0 0; 0 1 0; 0 0 1]
  iiwa_joint_2_OriginTransform : sm_lib/Frames and Transforms/Rigid Transform  TranslationMethod=Cartesian  TranslationStandardOffset=0  TranslationLengthUnit=m  TranslationStandardAxis=+Z  TranslationCartesianOffset=g_cm(1:3,4,7)'  TranslationROffset=0  TranslationROffsetUnits=m  TranslationZOffset=0  TranslationZOffsetUnits=m  TranslationThetaOffset=0  TranslationThetaOffsetUnits=deg  RotationMethod=RotationMatrix  RotationAngleUnits=deg  RotationStandardAxis=+Z  RotationAngle=0.0  RotationArbitraryAxis=[0 0 1]  FollAlignAxisA=+X  BaseAlignAxisA=+Y  FollAlignAxisB=+Y  BaseAlignAxisB=+Z  RotationSequenceAxes=BaseAxes  RotationSequence=XYZ  RotationSequenceAngles=[1.57079632679, 0, 3.14159265359]  RotationSequenceAnglesUnits=rad  RotationMatrix=g_cm(1:3,1:3,7)
  F : PMIOPort  Side=Left
  F1 : PMIOPort  Port=2  Side=Right
  connections:
  Base1/RConn1 -- VisualOriginTransform/RConn1
  F/RConn1 -- Inertia/RConn1 -- iiwa_joint_2_OriginTransform/RConn1 -- VisualOriginTransform/LConn1
  F1/RConn1 -- iiwa_joint_2_OriginTransform/LConn1

== system KUKAinv_Dynamics_coupled/Space Manipulator1/join//link 1 ==
  iiwa_joint_1 : sm_lib/Joints/Revolute Joint  JointMode=Normal  SenseConstraintForce=off  SenseConstraintForceX=off  SenseConstraintForceY=off  SenseConstraintForceZ=off  SenseConstraintTorque=off  SenseConstraintTorqueX=off  SenseConstraintTorqueY=off  SenseConstraintTorqueZ=off  SenseTotalForce=off  SenseTotalForceX=off  SenseTotalForceY=off  SenseTotalForceZ=off  SenseTotalTorque=off  SenseTotalTorqueX=off  SenseTotalTorqueY=off  SenseTotalTorqueZ=off  CompositeWrenchDir=FollowerOnBase  CompositeWrenchFrame=BaseFrame  EquilibriumPosition=0  EquilibriumPositionUnits=deg  SpringStiffness=0  SpringStiffnessUnits=N*m/deg  DampingCoefficient=0  DampingCoefficientUnits=kg*m^2/(rad*s)  TorqueActuationMode=InputTorque  MotionActuationMode=ComputedMotion  SensePosition=on  SenseVelocity=on  SenseAcceleration=on  SenseTorqueForce=off  SenseLowerLimitTorqueForce=off  SenseUpperLimitTorqueForce=off  LowerLimitSpecify=off  LowerLimitBound=-2.96705972839  LowerLimitBoundUnits=rad  LowerLimitStiffness=1e4  LowerLimitStiffnessUnits=N*m/deg  LowerLimitDamping=10  LowerLimitDampingUnits=N*m/(deg/s)  LowerLimitTransitionRegionWidth=0.1  LowerLimitTransitionRegionWidthUnits=deg  UpperLimitSpecify=off  UpperLimitBound=2.96705972839  UpperLimitBoundUnits=rad  UpperLimitStiffness=1e4  UpperLimitStiffnessUnits=N*m/deg  UpperLimitDamping=10  UpperLimitDampingUnits=N*m/(deg/s)  UpperLimitTransitionRegionWidth=0.1  UpperLimitTransitionRegionWidthUnits=deg  PositionTargetSpecify=on  PositionTargetPriority=High  PositionTargetValue=q_m(7)  PositionTargetValueUnits=rad  VelocityTargetSpecify=on  VelocityTargetPriority=High  VelocityTargetValue=q_dot_m(7)  VelocityTargetValueUnits=rad/s
  iiwa_link_1 : Subsystem
  b : PMIOPort  Side=Left
  f1 : PMIOPort  Port=2  Side=Left
  F1 : PMIOPort  Port=3  Side=Right
  q1 : PMIOPort  Port=4  Side=Right
  qd1 : PMIOPort  Port=5  Side=Right
  qdd1 : PMIOPort  Port=6  Side=Right
  connections:
  iiwa_link_1/LConn1 -- iiwa_joint_1/LConn1
  iiwa_joint_1/RConn1 -- b/RConn1
  iiwa_joint_1/RConn2 -- q1/RConn1
  f1/RConn1 -- iiwa_joint_1/LConn2
  iiwa_joint_1/RConn3 -- qd1/RConn1
  iiwa_joint_1/RConn4 -- qdd1/RConn1
  F1/RConn1 -- iiwa_link_1/RConn1

== system KUKAinv_Dynamics_coupled/Space Manipulator1/joint//link2 ==
  iiwa_joint_2 : sm_lib/Joints/Revolute Joint  JointMode=Normal  SenseConstraintForce=off  SenseConstraintForceX=off  SenseConstraintForceY=off  SenseConstraintForceZ=off  SenseConstraintTorque=off  SenseConstraintTorqueX=off  SenseConstraintTorqueY=off  SenseConstraintTorqueZ=off  SenseTotalForce=off  SenseTotalForceX=off  SenseTotalForceY=off  SenseTotalForceZ=off  SenseTotalTorque=off  SenseTotalTorqueX=off  SenseTotalTorqueY=off  SenseTotalTorqueZ=off  CompositeWrenchDir=FollowerOnBase  CompositeWrenchFrame=BaseFrame  EquilibriumPosition=0  EquilibriumPositionUnits=deg  SpringStiffness=0  SpringStiffnessUnits=N*m/deg  DampingCoefficient=0  DampingCoefficientUnits=kg*m^2/(rad*s)  TorqueActuationMode=InputTorque  MotionActuationMode=ComputedMotion  SensePosition=on  SenseVelocity=on  SenseAcceleration=on  SenseTorqueForce=off  SenseLowerLimitTorqueForce=off  SenseUpperLimitTorqueForce=off  LowerLimitSpecify=off  LowerLimitBound=-2.09439510239  LowerLimitBoundUnits=rad  LowerLimitStiffness=1e4  LowerLimitStiffnessUnits=N*m/deg  LowerLimitDamping=10  LowerLimitDampingUnits=N*m/(deg/s)  LowerLimitTransitionRegionWidth=0.1  LowerLimitTransitionRegionWidthUnits=deg  UpperLimitSpecify=off  UpperLimitBound=2.09439510239  UpperLimitBoundUnits=rad  UpperLimitStiffness=1e4  UpperLimitStiffnessUnits=N*m/deg  UpperLimitDamping=10  UpperLimitDampingUnits=N*m/(deg/s)  UpperLimitTransitionRegionWidth=0.1  UpperLimitTransitionRegionWidthUnits=deg  PositionTargetSpecify=on  PositionTargetPriority=High  PositionTargetValue=q_m(6)  PositionTargetValueUnits=rad  VelocityTargetSpecify=on  VelocityTargetPriority=High  VelocityTargetValue=q_dot_m(6)  VelocityTargetValueUnits=rad/s
  iiwa_link_2 : Subsystem
  b : PMIOPort  Side=Left
  F1 : PMIOPort  Port=2  Side=Right
  f2 : PMIOPort  Port=3  Side=Left
  q2 : PMIOPort  Port=4  Side=Right
  qd2 : PMIOPort  Port=5  Side=Right
  qdd2 : PMIOPort  Port=6  Side=Right
  connections:
  iiwa_joint_2/RConn3 -- qd2/RConn1
  iiwa_link_2/LConn1 -- iiwa_joint_2/LConn1
  F1/RConn1 -- iiwa_link_2/RConn1
  iiwa_joint_2/RConn4 -- qdd2/RConn1
  iiwa_joint_2/RConn1 -- b/RConn1
  f2/RConn1 -- iiwa_joint_2/LConn2
  iiwa_joint_2/RConn2 -- q2/RConn1

== system KUKAinv_Dynamics_coupled/Space Manipulator1/joint//link3 ==
  iiwa_joint_3 : sm_lib/Joints/Revolute Joint  JointMode=Normal  SenseConstraintForce=off  SenseConstraintForceX=off  SenseConstraintForceY=off  SenseConstraintForceZ=off  SenseConstraintTorque=off  SenseConstraintTorqueX=off  SenseConstraintTorqueY=off  SenseConstraintTorqueZ=off  SenseTotalForce=off  SenseTotalForceX=off  SenseTotalForceY=off  SenseTotalForceZ=off  SenseTotalTorque=off  SenseTotalTorqueX=off  SenseTotalTorqueY=off  SenseTotalTorqueZ=off  CompositeWrenchDir=FollowerOnBase  CompositeWrenchFrame=BaseFrame  EquilibriumPosition=0  EquilibriumPositionUnits=deg  SpringStiffness=0  SpringStiffnessUnits=N*m/deg  DampingCoefficient=0  DampingCoefficientUnits=kg*m^2/(rad*s)  TorqueActuationMode=InputTorque  MotionActuationMode=ComputedMotion  SensePosition=on  SenseVelocity=on  SenseAcceleration=on  SenseTorqueForce=off  SenseLowerLimitTorqueForce=off  SenseUpperLimitTorqueForce=off  LowerLimitSpecify=off  LowerLimitBound=-2.96705972839  LowerLimitBoundUnits=rad  LowerLimitStiffness=1e4  LowerLimitStiffnessUnits=N*m/deg  LowerLimitDamping=10  LowerLimitDampingUnits=N*m/(deg/s)  LowerLimitTransitionRegionWidth=0.1  LowerLimitTransitionRegionWidthUnits=deg  UpperLimitSpecify=off  UpperLimitBound=2.96705972839  UpperLimitBoundUnits=rad  UpperLimitStiffness=1e4  UpperLimitStiffnessUnits=N*m/deg  UpperLimitDamping=10  UpperLimitDampingUnits=N*m/(deg/s)  UpperLimitTransitionRegionWidth=0.1  UpperLimitTransitionRegionWidthUnits=deg  PositionTargetSpecify=on  PositionTargetPriority=High  PositionTargetValue=q_m(5)  PositionTargetValueUnits=rad  VelocityTargetSpecify=on  VelocityTargetPriority=High  VelocityTargetValue=q_dot_m(5)  VelocityTargetValueUnits=rad/s
  iiwa_link_3 : Subsystem
  b : PMIOPort  Side=Left
  F1 : PMIOPort  Port=2  Side=Right
  f3 : PMIOPort  Port=3  Side=Left
  q3 : PMIOPort  Port=4  Side=Right
  qd3 : PMIOPort  Port=5  Side=Right
  qdd3 : PMIOPort  Port=6  Side=Right
  connections:
  iiwa_link_3/LConn1 -- iiwa_joint_3/LConn1
  iiwa_joint_3/RConn4 -- qdd3/RConn1
  iiwa_joint_3/RConn3 -- qd3/RConn1
  iiwa_joint_3/RConn2 -- q3/RConn1
  F1/RConn1 -- iiwa_link_3/RConn1
  f3/RConn1 -- iiwa_joint_3/LConn2
  iiwa_joint_3/RConn1 -- b/RConn1

== system KUKAinv_Dynamics_coupled/Space Manipulator1/joint//link4 ==
  iiwa_joint_4 : sm_lib/Joints/Revolute Joint  JointMode=Normal  SenseConstraintForce=off  SenseConstraintForceX=off  SenseConstraintForceY=off  SenseConstraintForceZ=off  SenseConstraintTorque=off  SenseConstraintTorqueX=off  SenseConstraintTorqueY=off  SenseConstraintTorqueZ=off  SenseTotalForce=off  SenseTotalForceX=off  SenseTotalForceY=off  SenseTotalForceZ=off  SenseTotalTorque=off  SenseTotalTorqueX=off  SenseTotalTorqueY=off  SenseTotalTorqueZ=off  CompositeWrenchDir=FollowerOnBase  CompositeWrenchFrame=BaseFrame  EquilibriumPosition=0  EquilibriumPositionUnits=deg  SpringStiffness=0  SpringStiffnessUnits=N*m/deg  DampingCoefficient=0  DampingCoefficientUnits=kg*m^2/(rad*s)  TorqueActuationMode=InputTorque  MotionActuationMode=ComputedMotion  SensePosition=on  SenseVelocity=on  SenseAcceleration=on  SenseTorqueForce=off  SenseLowerLimitTorqueForce=off  SenseUpperLimitTorqueForce=off  LowerLimitSpecify=off  LowerLimitBound=-2.09439510239  LowerLimitBoundUnits=rad  LowerLimitStiffness=1e4  LowerLimitStiffnessUnits=N*m/deg  LowerLimitDamping=10  LowerLimitDampingUnits=N*m/(deg/s)  LowerLimitTransitionRegionWidth=0.1  LowerLimitTransitionRegionWidthUnits=deg  UpperLimitSpecify=off  UpperLimitBound=2.09439510239  UpperLimitBoundUnits=rad  UpperLimitStiffness=1e4  UpperLimitStiffnessUnits=N*m/deg  UpperLimitDamping=10  UpperLimitDampingUnits=N*m/(deg/s)  UpperLimitTransitionRegionWidth=0.1  UpperLimitTransitionRegionWidthUnits=deg  PositionTargetSpecify=on  PositionTargetPriority=High  PositionTargetValue=q_m(4)  PositionTargetValueUnits=rad  VelocityTargetSpecify=on  VelocityTargetPriority=High  VelocityTargetValue=q_dot_m(4)  VelocityTargetValueUnits=rad/s
  iiwa_link_4 : Subsystem
  b : PMIOPort  Side=Left
  F1 : PMIOPort  Port=2  Side=Right
  f4 : PMIOPort  Port=3  Side=Left
  q4 : PMIOPort  Port=4  Side=Right
  qd4 : PMIOPort  Port=5  Side=Right
  qdd4 : PMIOPort  Port=6  Side=Right
  connections:
  iiwa_link_4/LConn1 -- iiwa_joint_4/LConn1
  iiwa_joint_4/RConn3 -- qd4/RConn1
  f4/RConn1 -- iiwa_joint_4/LConn2
  F1/RConn1 -- iiwa_link_4/RConn1
  iiwa_joint_4/RConn2 -- q4/RConn1
  iiwa_joint_4/RConn1 -- b/RConn1
  iiwa_joint_4/RConn4 -- qdd4/RConn1

== system KUKAinv_Dynamics_coupled/Space Manipulator1/joint//link5 ==
  iiwa_joint_5 : sm_lib/Joints/Revolute Joint  JointMode=Normal  SenseConstraintForce=off  SenseConstraintForceX=off  SenseConstraintForceY=off  SenseConstraintForceZ=off  SenseConstraintTorque=off  SenseConstraintTorqueX=off  SenseConstraintTorqueY=off  SenseConstraintTorqueZ=off  SenseTotalForce=off  SenseTotalForceX=off  SenseTotalForceY=off  SenseTotalForceZ=off  SenseTotalTorque=off  SenseTotalTorqueX=off  SenseTotalTorqueY=off  SenseTotalTorqueZ=off  CompositeWrenchDir=FollowerOnBase  CompositeWrenchFrame=BaseFrame  EquilibriumPosition=0  EquilibriumPositionUnits=rad  SpringStiffness=0  SpringStiffnessUnits=N*m/rad  DampingCoefficient=0  DampingCoefficientUnits=kg*m^2/(rad*s)  TorqueActuationMode=InputTorque  MotionActuationMode=ComputedMotion  SensePosition=on  SenseVelocity=on  SenseAcceleration=on  SenseTorqueForce=off  SenseLowerLimitTorqueForce=off  SenseUpperLimitTorqueForce=off  LowerLimitSpecify=off  LowerLimitBound=-2.96705972839  LowerLimitBoundUnits=rad  LowerLimitStiffness=1e4  LowerLimitStiffnessUnits=N*m/deg  LowerLimitDamping=10  LowerLimitDampingUnits=N*m/(deg/s)  LowerLimitTransitionRegionWidth=0.1  LowerLimitTransitionRegionWidthUnits=deg  UpperLimitSpecify=off  UpperLimitBound=2.96705972839  UpperLimitBoundUnits=rad  UpperLimitStiffness=1e4  UpperLimitStiffnessUnits=N*m/deg  UpperLimitDamping=10  UpperLimitDampingUnits=N*m/(deg/s)  UpperLimitTransitionRegionWidth=0.1  UpperLimitTransitionRegionWidthUnits=deg  PositionTargetSpecify=on  PositionTargetPriority=High  PositionTargetValue=q_m(3)  PositionTargetValueUnits=rad  VelocityTargetSpecify=on  VelocityTargetPriority=High  VelocityTargetValue=q_dot_m(3)  VelocityTargetValueUnits=rad/s
  iiwa_link_5 : Subsystem
  b : PMIOPort  Side=Left
  F1 : PMIOPort  Port=2  Side=Right
  f5 : PMIOPort  Port=3  Side=Left
  q5 : PMIOPort  Port=4  Side=Right
  qd5 : PMIOPort  Port=5  Side=Right
  qdd5 : PMIOPort  Port=6  Side=Right
  connections:
  iiwa_joint_5/RConn1 -- b/RConn1
  iiwa_joint_5/RConn2 -- q5/RConn1
  iiwa_joint_5/RConn4 -- qdd5/RConn1
  iiwa_link_5/LConn1 -- iiwa_joint_5/LConn1
  iiwa_joint_5/RConn3 -- qd5/RConn1
  f5/RConn1 -- iiwa_joint_5/LConn2
  F1/RConn1 -- iiwa_link_5/RConn1

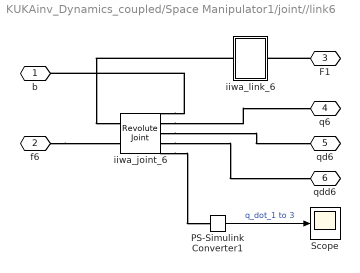
== system KUKAinv_Dynamics_coupled/Space Manipulator1/joint//link6 ==
  PS-Simulink Converter1 : nesl_utility/PS-Simulink Converter  PhysicalDomain=network_engine_domain  SubClassName=ps_output  LeftPortType=input  RightPortType=output  PseudoPeriodic=off  Frequencies=[]  Unit=inherit  AffineConversion=off
      settings: SourceProductBaseCode=PW,SS
  Scope : Scope
  iiwa_joint_6 : sm_lib/Joints/Revolute Joint  JointMode=Normal  SenseConstraintForce=off  SenseConstraintForceX=off  SenseConstraintForceY=off  SenseConstraintForceZ=off  SenseConstraintTorque=off  SenseConstraintTorqueX=off  SenseConstraintTorqueY=off  SenseConstraintTorqueZ=off  SenseTotalForce=off  SenseTotalForceX=off  SenseTotalForceY=off  SenseTotalForceZ=off  SenseTotalTorque=off  SenseTotalTorqueX=off  SenseTotalTorqueY=off  SenseTotalTorqueZ=off  CompositeWrenchDir=FollowerOnBase  CompositeWrenchFrame=BaseFrame  EquilibriumPosition=0  EquilibriumPositionUnits=rad  SpringStiffness=0  SpringStiffnessUnits=N*m/rad  DampingCoefficient=0  DampingCoefficientUnits=kg*m^2/(rad*s)  TorqueActuationMode=InputTorque  MotionActuationMode=ComputedMotion  SensePosition=on  SenseVelocity=on  SenseAcceleration=on  SenseTorqueForce=on  SenseLowerLimitTorqueForce=off  SenseUpperLimitTorqueForce=off  LowerLimitSpecify=off  LowerLimitBound=-2.09439510239  LowerLimitBoundUnits=rad  LowerLimitStiffness=1e4  LowerLimitStiffnessUnits=N*m/deg  LowerLimitDamping=10  LowerLimitDampingUnits=N*m/(deg/s)  LowerLimitTransitionRegionWidth=0.1  LowerLimitTransitionRegionWidthUnits=deg  UpperLimitSpecify=off  UpperLimitBound=2.09439510239  UpperLimitBoundUnits=rad  UpperLimitStiffness=1e4  UpperLimitStiffnessUnits=N*m/deg  UpperLimitDamping=10  UpperLimitDampingUnits=N*m/(deg/s)  UpperLimitTransitionRegionWidth=0.1  UpperLimitTransitionRegionWidthUnits=deg  PositionTargetSpecify=on  PositionTargetPriority=High  PositionTargetValue=q_m(2)  PositionTargetValueUnits=rad  VelocityTargetSpecify=on  VelocityTargetPriority=High  VelocityTargetValue=q_dot_m(2)  VelocityTargetValueUnits=rad/s
  iiwa_link_6 : Subsystem
  b : PMIOPort  Side=Left
  f6 : PMIOPort  Port=2  Side=Left
  F1 : PMIOPort  Port=3  Side=Right
  q6 : PMIOPort  Port=4  Side=Right
  qd6 : PMIOPort  Port=5  Side=Right
  qdd6 : PMIOPort  Port=6  Side=Right
  wires:
  PS-Simulink Converter1/1 -> Scope/1  "q_dot_1 to 3"
  connections:
  iiwa_link_6/LConn1 -- iiwa_joint_6/LConn1
  iiwa_joint_6/RConn1 -- b/RConn1
  F1/RConn1 -- iiwa_link_6/RConn1
  f6/RConn1 -- iiwa_joint_6/LConn2
  iiwa_joint_6/RConn4 -- qdd6/RConn1
  iiwa_joint_6/RConn3 -- qd6/RConn1
  iiwa_joint_6/RConn2 -- q6/RConn1
  iiwa_joint_6/RConn5 -- PS-Simulink Converter1/LConn1

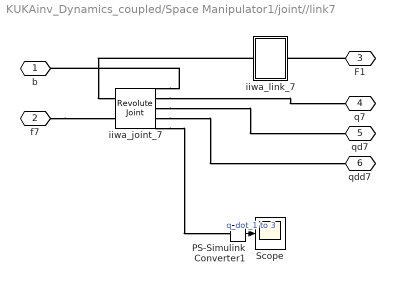
== system KUKAinv_Dynamics_coupled/Space Manipulator1/joint//link7 ==
  PS-Simulink Converter1 : nesl_utility/PS-Simulink Converter  PhysicalDomain=network_engine_domain  SubClassName=ps_output  LeftPortType=input  RightPortType=output  PseudoPeriodic=off  Frequencies=[]  Unit=inherit  AffineConversion=off
      settings: SourceProductBaseCode=PW,SS
  Scope : Scope
  iiwa_joint_7 : sm_lib/Joints/Revolute Joint  JointMode=Normal  SenseConstraintForce=off  SenseConstraintForceX=off  SenseConstraintForceY=off  SenseConstraintForceZ=off  SenseConstraintTorque=off  SenseConstraintTorqueX=off  SenseConstraintTorqueY=off  SenseConstraintTorqueZ=off  SenseTotalForce=off  SenseTotalForceX=off  SenseTotalForceY=off  SenseTotalForceZ=off  SenseTotalTorque=off  SenseTotalTorqueX=off  SenseTotalTorqueY=off  SenseTotalTorqueZ=off  CompositeWrenchDir=FollowerOnBase  CompositeWrenchFrame=BaseFrame  EquilibriumPosition=0  EquilibriumPositionUnits=rad  SpringStiffness=0  SpringStiffnessUnits=N*m/rad  DampingCoefficient=0  DampingCoefficientUnits=kg*m^2/(rad*s)  TorqueActuationMode=InputTorque  MotionActuationMode=ComputedMotion  SensePosition=on  SenseVelocity=on  SenseAcceleration=on  SenseTorqueForce=on  SenseLowerLimitTorqueForce=off  SenseUpperLimitTorqueForce=off  LowerLimitSpecify=off  LowerLimitBound=-3.05432619099  LowerLimitBoundUnits=rad  LowerLimitStiffness=1e4  LowerLimitStiffnessUnits=N*m/deg  LowerLimitDamping=10  LowerLimitDampingUnits=N*m/(deg/s)  LowerLimitTransitionRegionWidth=0.1  LowerLimitTransitionRegionWidthUnits=deg  UpperLimitSpecify=off  UpperLimitBound=3.05432619099  UpperLimitBoundUnits=rad  UpperLimitStiffness=1e4  UpperLimitStiffnessUnits=N*m/deg  UpperLimitDamping=10  UpperLimitDampingUnits=N*m/(deg/s)  UpperLimitTransitionRegionWidth=0.1  UpperLimitTransitionRegionWidthUnits=deg  PositionTargetSpecify=on  PositionTargetPriority=High  PositionTargetValue=q_m(1)  PositionTargetValueUnits=rad  VelocityTargetSpecify=on  VelocityTargetPriority=High  VelocityTargetValue=q_dot_m(1)  VelocityTargetValueUnits=rad/s
  iiwa_link_7 : Subsystem
  b : PMIOPort  Side=Left
  f7 : PMIOPort  Port=2  Side=Left
  F1 : PMIOPort  Port=3  Side=Right
  q7 : PMIOPort  Port=4  Side=Right
  qd7 : PMIOPort  Port=5  Side=Right
  qdd7 : PMIOPort  Port=6  Side=Right
  wires:
  PS-Simulink Converter1/1 -> Scope/1  "q_dot_1 to 3"
  connections:
  iiwa_link_7/LConn1 -- iiwa_joint_7/LConn1
  iiwa_joint_7/RConn4 -- qdd7/RConn1
  iiwa_joint_7/RConn2 -- q7/RConn1
  iiwa_joint_7/RConn3 -- qd7/RConn1
  f7/RConn1 -- iiwa_joint_7/LConn2
  F1/RConn1 -- iiwa_link_7/RConn1
  iiwa_joint_7/RConn1 -- b/RConn1
  iiwa_joint_7/RConn5 -- PS-Simulink Converter1/LConn1

== system KUKAinv_Dynamics_coupled/time-dependent variables' calculations/A_connection ==
  M0 : Inport
  M0m : Inport  Port=2
  Divide : Product  Inputs=/*  Multiplication=Matrix(*)
  A : Outport
  wires:
  Divide/1 -> A/1
  M0/1 -> Divide/1
  M0m/1 -> Divide/2
